simulink model "sampleModel1857_1_sub_sub"  (R2023a)
settings: Solver=VariableStepAuto  StartTime=0.0  StopTime=10.0  RelTol=1e-3
libraries: hdlsllib x4, simulink x2
settings Model: Creator=user1  LastModifiedBy=user1

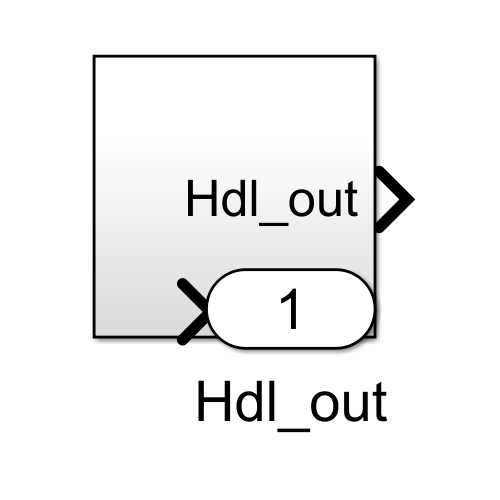
[thumbnail: Simulink's stored preview of the top-level diagram]
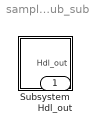
== system sampleModel1857_1_sub_sub ==
  Subsystem : Subsystem
  Hdl_out : Outport  OutDataTypeStr=uint8

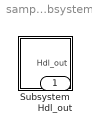
== system sampleModel1857_1_sub_sub/Subsystem ==
  Subsystem : Subsystem
  Hdl_out : Outport  OutDataTypeStr=uint8

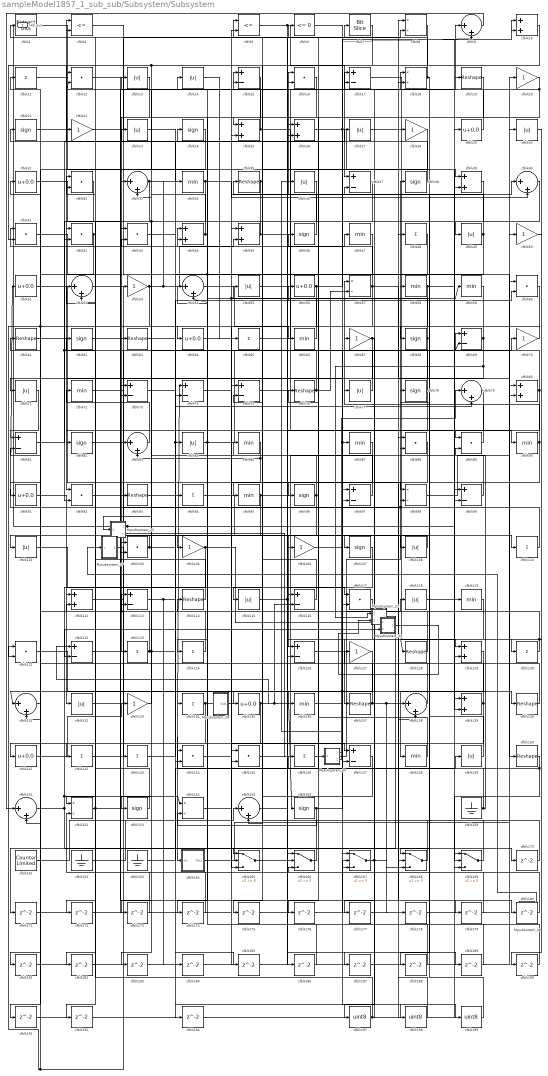
== system sampleModel1857_1_sub_sub/Subsystem/Subsystem ==
  Mysubsystem_10 : Subsystem  TreatAsAtomicUnit=on  RTWFcnName=Mysubsystem_10
      settings: RTWFcnNameOpts=User specified  RTWFileNameOpts=Use function name
  Mysubsystem_22 : Subsystem  TreatAsAtomicUnit=on  RTWFcnName=Mysubsystem_22
      settings: RTWFcnNameOpts=User specified  RTWFileNameOpts=Use function name
  Mysubsystem_23 : Subsystem  TreatAsAtomicUnit=on  RTWFcnName=Mysubsystem_23
      settings: RTWFcnNameOpts=User specified  RTWFileNameOpts=Use function name
  Mysubsystem_31 : Subsystem  TreatAsAtomicUnit=on  RTWFcnName=Mysubsystem_31
      settings: RTWFcnNameOpts=User specified  RTWFileNameOpts=Use function name
  Mysubsystem_37 : Subsystem  TreatAsAtomicUnit=on  RTWFcnName=Mysubsystem_37
      settings: RTWFcnNameOpts=User specified  RTWFileNameOpts=Use function name
  Mysubsystem_39 : Subsystem  TreatAsAtomicUnit=on  RTWFcnName=Mysubsystem_39
      settings: RTWFcnNameOpts=User specified  RTWFileNameOpts=Use function name
  Mysubsystem_40 : Subsystem  TreatAsAtomicUnit=on  RTWFcnName=Mysubsystem_40
      settings: RTWFcnNameOpts=User specified  RTWFileNameOpts=Use function name
  cfblk1 : simulink/Logic and Bit Operations/Extract Bits  bitsToExtract=Upper half  numBits=8  bitIdxRange=[0 7]  outScalingMode=Preserve fixed-point scaling
      settings: LibrarySourceBlock=|
      | hdlsllib/Logic and Bit
      | Operations/Extract Bits
  cfblk{10,25..26,39,44..45,80,112,129,139} (10 alike) : Sum  OutDataTypeStr=uint8
  cfblk{13..14,23,27,30,36,49,55,71,77,84,101,108,115,118,132,149} (17 alike) : Abs  OutDataTypeStr=uint8  SaturateOnIntegerOverflow=off
  cfblk{12,16,32,41..43,60,88..89,92,103,117,121,144..145} (15 alike) : DotProduct  OutDataTypeStr=uint8
  cfblk{20,22,28,50,53,67,70,104,106,127,133} (11 alike) : Gain  OutDataTypeStr=uint8
  cfblk{21,24,38,46,62,68,78,82,96,107,153,156} (12 alike) : Signum
  cfblk{11,48,65,94,110,123..124,130,134,142..143,146} (12 alike) : Sum  Inputs=+  OutDataTypeStr=uint8
  cfblk{15,17,37,69,73..75,81,97,99,113,116,122,126,147} (15 alike) : Sum  Inputs=+-  OutDataTypeStr=uint8
  cfblk{19,35,61,63,76,93,114,128,137,140,150} (11 alike) : Reshape
  cfblk{34,47,58..59,66,72,85,87,90,95,119,136,148} (13 alike) : MinMax  OutDataTypeStr=uint8
  cfblk{9,33,40,52,54,79,83,131,138,151,155} (11 alike) : Sum  Inputs=|++  OutDataTypeStr=uint8
  cfblk{29,31,51,56,64,91,135,141} (8 alike) : Bias  Bias=0.0  SaturateOnIntegerOverflow=off
  cfblk{8,18,57,98,152,154} (6 alike) : Product  Inputs=*/  OutDataTypeStr=uint8  RndMeth=Zero  SaturateOnIntegerOverflow=on
  cfblk159 : Ground
  cfblk161 : hdlsllib/Sources/Counter Limited  uplimit=7  tsamp=-1
  cfblk162 : Ground
  cfblk163 : Ground
  cfblk164 : Subsystem
      settings: LibrarySourceBlock=|
      | hdlsllib/Ports &
      | Subsystems/Subsystem
  cfblk{165..169} (5 alike) : Switch  OutDataTypeStr=uint8  SaturateOnIntegerOverflow=off  InputSameDT=off
  cfblk{170..192,194} (24 alike) : Delay  SampleTime=1
  cfblk197 : DataTypeConversion  OutDataTypeStr=uint8  SaturateOnIntegerOverflow=off  RndMeth=Floor
  cfblk198 : DataTypeConversion  OutDataTypeStr=uint8  SaturateOnIntegerOverflow=off  RndMeth=Floor
  cfblk199 : DataTypeConversion  OutDataTypeStr=uint8  SaturateOnIntegerOverflow=off  RndMeth=Floor
  cfblk2 : RelationalOperator  Operator=<=  OutDataTypeStr=boolean  InputSameDT=off
  cfblk5 : RelationalOperator  Operator=<=  OutDataTypeStr=boolean  InputSameDT=off
  cfblk6 : hdlsllib/Logic and Bit Operations/Compare To Zero  relop=<=  OutDataTypeStr=uint8
  cfblk7 : hdlsllib/Logic and Bit Operations/Bit Slice  lidx=7  ridx=0
  Hdl_out : Outport  OutDataTypeStr=uint8
  wires:
  Mysubsystem_40/1(Out1) -> Mysubsystem_37/1(u)
  Mysubsystem_39/1(Out1) -> cfblk122/1
  Mysubsystem_37/1(Out1) -> cfblk121/1, cfblk11/1
  Mysubsystem_31/1(Out1) -> Mysubsystem_22/2(In2)
  Mysubsystem_23/2(y) -> Mysubsystem_10/1(In1)
  Mysubsystem_23/1(Out1) -> cfblk129/2, Hdl_out/1
  Mysubsystem_22/1(Out1) -> cfblk171/1
  Mysubsystem_10/2(Out2) -> cfblk79/1
  Mysubsystem_10/1(Out1) -> cfblk36/1
  cfblk199/1 -> cfblk88/2
  cfblk198/1 -> cfblk88/1
  cfblk23/1 -> cfblk198/1
  cfblk197/1 -> cfblk22/1, cfblk127/1
  cfblk194/1 -> cfblk28/1
  cfblk63/1 -> cfblk194/1
  cfblk192/1 -> cfblk169/1
  cfblk191/1 -> cfblk138/2
  cfblk190/1 -> cfblk99/1
  cfblk50/1 -> cfblk190/1
  cfblk189/1 -> cfblk54/1
  cfblk106/1 -> cfblk189/1
  cfblk188/1 -> cfblk75/1
  cfblk187/1 -> cfblk18/2
  cfblk186/1 -> cfblk166/1
  cfblk165/1 -> cfblk186/1
  cfblk185/1 -> cfblk26/2
  cfblk184/1 -> cfblk25/2
  cfblk183/1 -> cfblk169/3
  cfblk182/1 -> cfblk45/1
  cfblk79/1 -> cfblk182/1
  cfblk181/1 -> cfblk60/1
  cfblk180/1 -> cfblk152/2
  cfblk179/1 -> cfblk166/3
  cfblk12/1 -> cfblk179/1
  cfblk178/1 -> cfblk39/2
  cfblk177/1 -> cfblk17/2
  cfblk176/1 -> cfblk167/2
  cfblk175/1 -> cfblk80/1
  cfblk147/1 -> cfblk175/1
  cfblk174/1 -> cfblk2/2
  cfblk173/1 -> cfblk52/1
  cfblk172/1 -> cfblk73/2
  cfblk171/1 -> cfblk145/1
  cfblk170/1 -> cfblk1/1
  cfblk74/1 -> cfblk170/1
  cfblk7/1 -> cfblk155/2
  cfblk116/1 -> cfblk15/1
  cfblk93/1 -> cfblk98/1
  cfblk85/1 -> cfblk145/2, cfblk83/2
  cfblk99/1 -> cfblk78/1
  cfblk161/1 -> cfblk5/2
  cfblk167/1 -> cfblk67/1, cfblk178/1
  cfblk76/1 -> cfblk55/1, cfblk57/2
  cfblk69/1 -> Mysubsystem_22/1(In1), cfblk191/1, cfblk68/1
  cfblk34/1 -> cfblk74/2, cfblk40/2
  cfblk67/1 -> cfblk176/1, cfblk177/1
  cfblk56/1 -> cfblk10/2, cfblk165/2
  cfblk18/1 -> cfblk5/1, cfblk168/1
  cfblk30/1 -> cfblk130/1
  cfblk124/1 -> cfblk31/1, cfblk113/1
  cfblk10/1 -> cfblk33/1, cfblk41/2
  cfblk80/1 -> cfblk13/1, cfblk172/1
  cfblk101/1 -> cfblk117/1
  cfblk81/1 -> cfblk27/1, cfblk69/2
  cfblk83/1 -> cfblk62/1
  cfblk132/1 -> cfblk83/1
  cfblk39/1 -> cfblk49/1
  cfblk87/1 -> cfblk165/1
  cfblk113/1 -> cfblk184/1, cfblk185/1
  cfblk152/1 -> cfblk73/1, cfblk192/1
  cfblk60/1 -> cfblk104/1
  cfblk48/1 -> cfblk144/2, cfblk174/1
  cfblk140/1 -> cfblk61/1
  cfblk151/1 -> Mysubsystem_31/2(In2), cfblk154/1, cfblk165/3
  cfblk19/1 -> cfblk103/2
  cfblk1/1 -> cfblk39/1
  cfblk54/1 -> cfblk106/1
  cfblk164/1(Out1) -> cfblk50/1
  cfblk37/1 -> cfblk42/2
  cfblk77/1 -> cfblk46/1
  cfblk38/1 -> cfblk2/1
  cfblk73/1 -> cfblk60/2
  cfblk131/1 -> cfblk81/2
  cfblk115/1 -> cfblk7/1, cfblk168/2
  cfblk61/1 -> cfblk167/1
  cfblk127/1 -> cfblk131/1, cfblk147/2
  cfblk58/1 -> cfblk10/1, cfblk71/1
  cfblk28/1 -> cfblk135/1
  cfblk46/1 -> cfblk35/1
  cfblk108/1 -> cfblk103/1
  cfblk154/1 -> cfblk59/1, cfblk40/1
  cfblk144/1 -> cfblk147/1
  cfblk78/1 -> cfblk153/1, cfblk24/1
  cfblk122/1 -> cfblk17/1
  cfblk138/1 -> cfblk6/1
  cfblk15/1 -> cfblk64/1
  cfblk133/1 -> cfblk23/1
  cfblk32/1 -> cfblk92/2
  cfblk68/1 -> cfblk21/1, cfblk167/3
  cfblk71/1 -> cfblk81/1
  cfblk29/1 -> cfblk19/1
  cfblk47/1 -> cfblk116/1
  cfblk36/1 -> Mysubsystem_23/1(In1), cfblk113/2
  cfblk42/1 -> cfblk112/1, cfblk181/1
  cfblk141/1 -> cfblk133/1
  cfblk112/1 -> cfblk48/1
  cfblk72/1 -> cfblk30/1
  cfblk92/1 -> cfblk136/1
  cfblk166/1 -> cfblk41/1
  cfblk25/1 -> cfblk150/1, cfblk15/2
  cfblk136/1 -> cfblk140/1
  cfblk123/1 -> cfblk79/2, cfblk183/1, cfblk32/2
  cfblk2/1 -> cfblk99/2
  cfblk168/1 -> cfblk44/2
  cfblk143/1 -> cfblk56/1
  cfblk53/1 -> cfblk121/2, cfblk91/1, cfblk45/2, cfblk34/1
  cfblk118/1 -> cfblk139/1
  cfblk16/1 -> cfblk25/1
  cfblk41/1 -> cfblk53/1
  cfblk163/1 -> cfblk146/1
  cfblk35/1 -> cfblk115/1, cfblk134/1
  cfblk20/1 -> cfblk96/1, cfblk12/2
  cfblk82/1 -> cfblk97/2
  cfblk103/1 -> cfblk101/1, cfblk117/2
  cfblk59/1 -> cfblk124/1
  cfblk153/1 -> cfblk72/1
  cfblk88/1 -> cfblk197/1
  cfblk64/1 -> cfblk108/1
  cfblk156/1 -> cfblk70/1, cfblk154/2
  cfblk6/1 -> cfblk87/1, cfblk199/1
  cfblk149/1 -> cfblk37/2
  cfblk11/1 -> cfblk143/1
  cfblk65/1 -> cfblk9/1
  cfblk44/1 -> cfblk144/1, cfblk12/1
  cfblk70/1 -> cfblk63/1
  cfblk62/1 -> cfblk138/1
  cfblk22/1 -> cfblk8/2
  cfblk130/1 -> cfblk52/2, cfblk128/1
  cfblk121/1 -> cfblk164/1(In1)
  cfblk13/1 -> cfblk93/1
  cfblk45/1 -> cfblk97/1, cfblk43/1
  cfblk31/1 -> cfblk123/1
  cfblk119/1 -> cfblk166/2
  cfblk137/1 -> cfblk168/3, cfblk180/1, cfblk75/2
  cfblk169/1 -> cfblk85/1
  cfblk162/1 -> cfblk155/1
  cfblk97/1 -> cfblk44/1
  cfblk155/1 -> cfblk149/1
  cfblk57/1 -> cfblk80/2, cfblk43/2, cfblk131/2
  cfblk40/1 -> cfblk82/1
  cfblk75/1 -> cfblk90/1
  cfblk129/1 -> cfblk148/1
  cfblk21/1 -> cfblk94/1
  cfblk98/1 -> cfblk20/1
  cfblk26/1 -> cfblk119/1, cfblk9/2
  cfblk134/1 -> cfblk151/2, cfblk18/1
  cfblk9/1 -> cfblk151/1
  cfblk84/1 -> cfblk29/1, cfblk54/2
  cfblk90/1 -> cfblk77/1, cfblk188/1
  cfblk139/1 -> cfblk112/2, cfblk173/1
  cfblk107/1 -> cfblk126/2
  cfblk117/1 -> cfblk137/1
  cfblk51/1 -> cfblk95/1
  cfblk95/1 -> cfblk152/1, cfblk47/1
  cfblk91/1 -> cfblk132/1
  cfblk27/1 -> cfblk8/1
  cfblk96/1 -> cfblk126/1, cfblk33/2
  cfblk89/1 -> cfblk57/1
  cfblk146/1 -> cfblk58/1
  cfblk94/1 -> cfblk107/1
  cfblk114/1 -> cfblk32/1
  cfblk43/1 -> cfblk84/1, cfblk139/2
  cfblk24/1 -> cfblk141/1
  cfblk5/1 -> cfblk37/1, cfblk187/1
  cfblk104/1 -> Mysubsystem_31/1(In1), cfblk122/2
  cfblk135/1 -> cfblk156/1, cfblk116/2, cfblk142/1
  cfblk66/1 -> cfblk14/1
  cfblk52/1 -> cfblk110/1
  cfblk110/1 -> cfblk51/1, cfblk98/2
  cfblk49/1 -> cfblk16/2, cfblk66/1
  cfblk148/1 -> cfblk76/1
  cfblk142/1 -> cfblk69/1
  cfblk145/1 -> cfblk38/1
  cfblk128/1 -> cfblk114/1
  cfblk159/1 -> cfblk16/1, cfblk89/2
  cfblk55/1 -> cfblk89/1
  cfblk8/1 -> cfblk42/1
  cfblk126/1 -> cfblk118/1
  cfblk150/1 -> cfblk74/1, cfblk169/2
  cfblk33/1 -> cfblk92/1, cfblk26/1
  cfblk17/1 -> cfblk129/1
  cfblk14/1 -> cfblk65/1

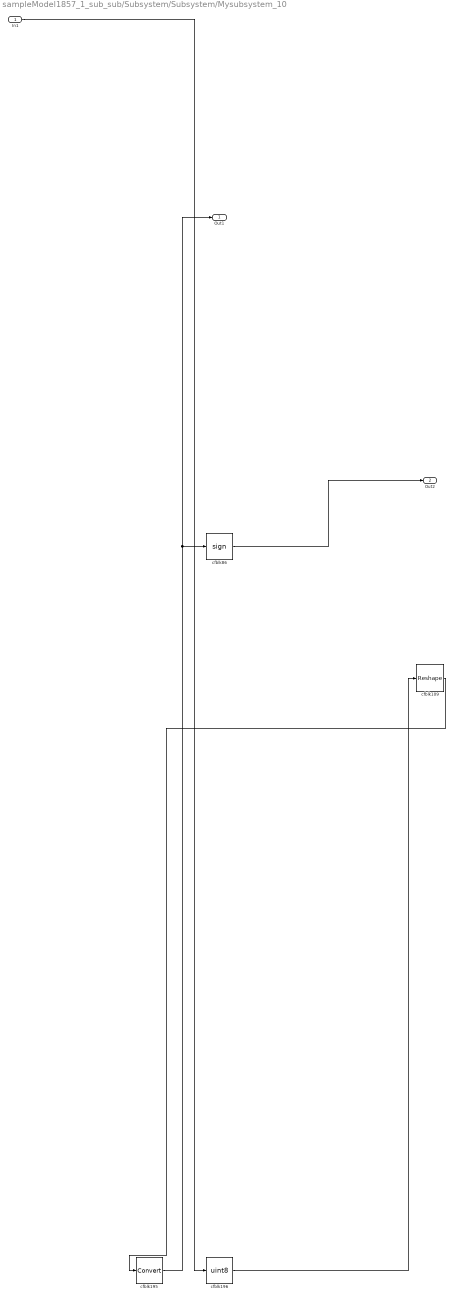
== system sampleModel1857_1_sub_sub/Subsystem/Subsystem/Mysubsystem_10 ==
  In1 : Inport
  cfblk109 : Reshape
  cfblk195 : DataTypeConversion  SaturateOnIntegerOverflow=off  RndMeth=Floor
  cfblk196 : DataTypeConversion  OutDataTypeStr=uint8  SaturateOnIntegerOverflow=off  RndMeth=Floor
  cfblk86 : Signum
  Out1 : Outport
  Out2 : Outport  Port=2
  wires:
  cfblk86/1 -> Out2/1
  cfblk109/1 -> cfblk195/1
  cfblk195/1 -> Out1/1, cfblk86/1
  cfblk196/1 -> cfblk109/1
  In1/1 -> cfblk196/1

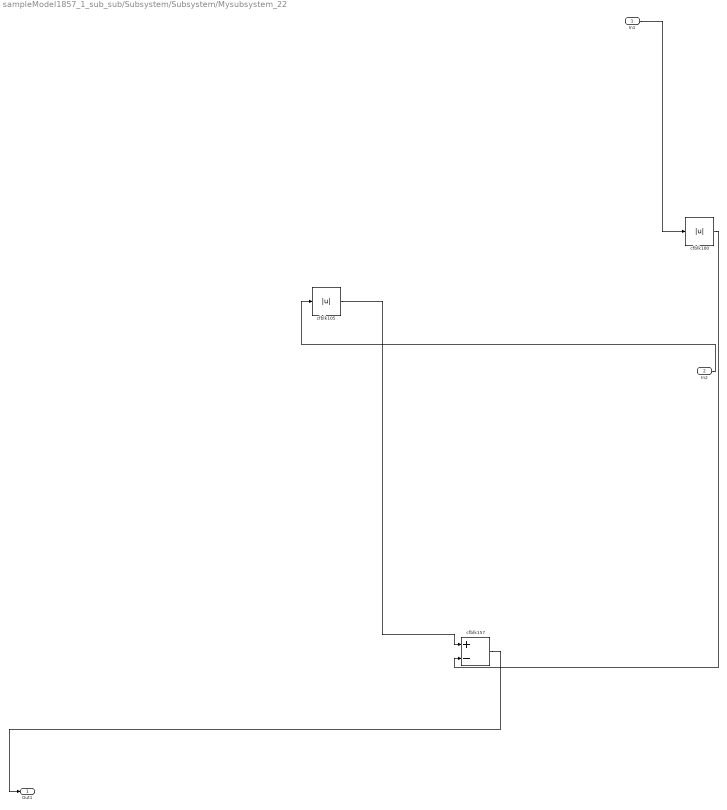
== system sampleModel1857_1_sub_sub/Subsystem/Subsystem/Mysubsystem_22 ==
  In1 : Inport
  In2 : Inport  Port=2
  cfblk100 : Abs  SaturateOnIntegerOverflow=off
  cfblk105 : Abs  SaturateOnIntegerOverflow=off
  cfblk157 : Sum  Inputs=+-
  Out1 : Outport
  wires:
  cfblk105/1 -> cfblk157/1
  In2/1 -> cfblk105/1
  cfblk100/1 -> cfblk157/2
  cfblk157/1 -> Out1/1
  In1/1 -> cfblk100/1

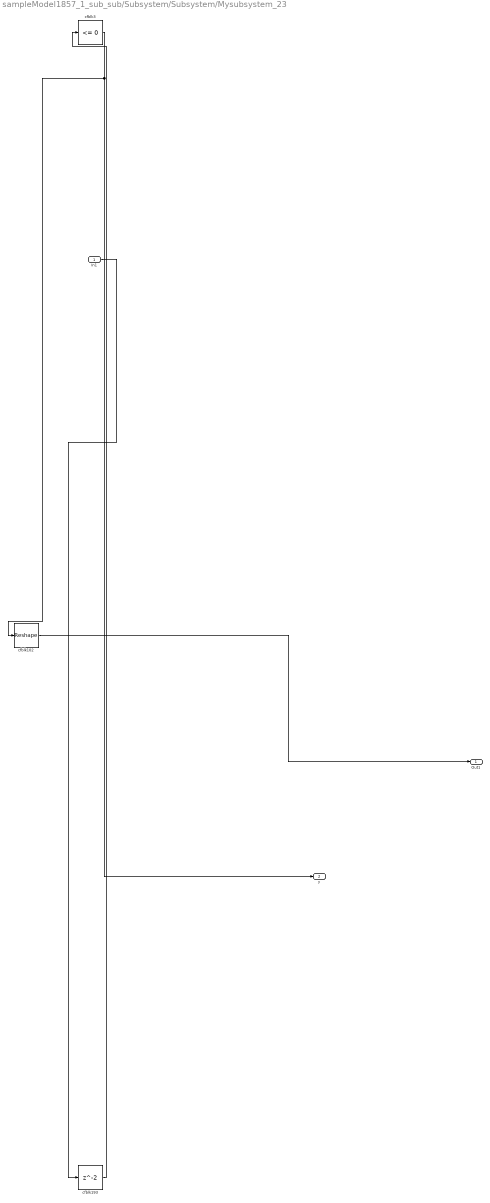
== system sampleModel1857_1_sub_sub/Subsystem/Subsystem/Mysubsystem_23 ==
  In1 : Inport
  cfblk102 : Reshape
  cfblk193 : Delay  SampleTime=1
  cfblk3 : hdlsllib/Logic and Bit Operations/Compare To Zero  relop=<=  OutDataTypeStr=boolean
  Out1 : Outport
  y : Outport  Port=2
  wires:
  cfblk193/1 -> cfblk3/1
  cfblk3/1 -> y/1, cfblk102/1
  cfblk102/1 -> Out1/1
  In1/1 -> cfblk193/1

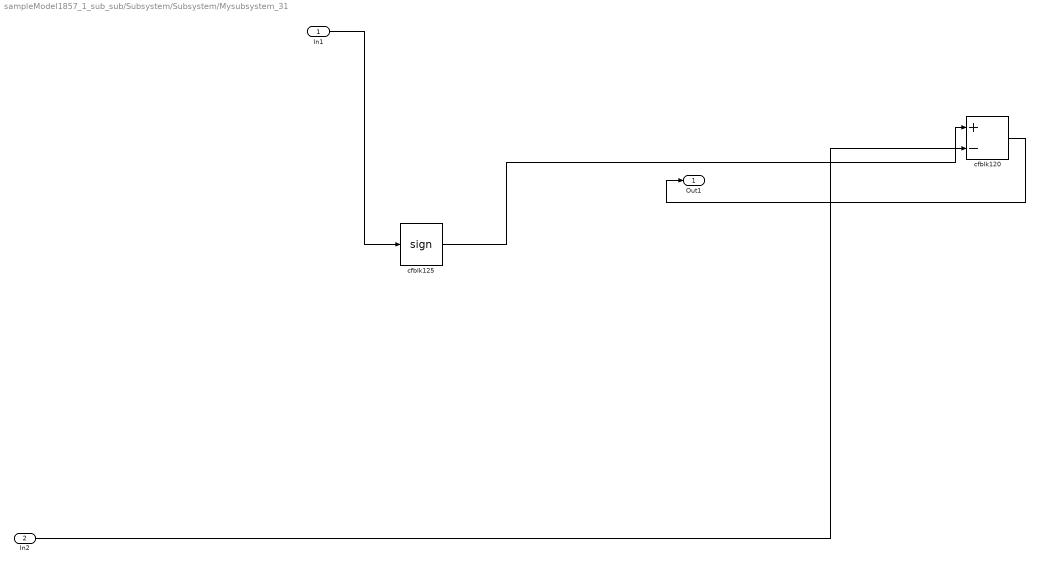
== system sampleModel1857_1_sub_sub/Subsystem/Subsystem/Mysubsystem_31 ==
  In1 : Inport
  In2 : Inport  Port=2
  cfblk120 : Sum  Inputs=+-
  cfblk125 : Signum
  Out1 : Outport
  wires:
  cfblk125/1 -> cfblk120/1
  In2/1 -> cfblk120/2
  In1/1 -> cfblk125/1
  cfblk120/1 -> Out1/1

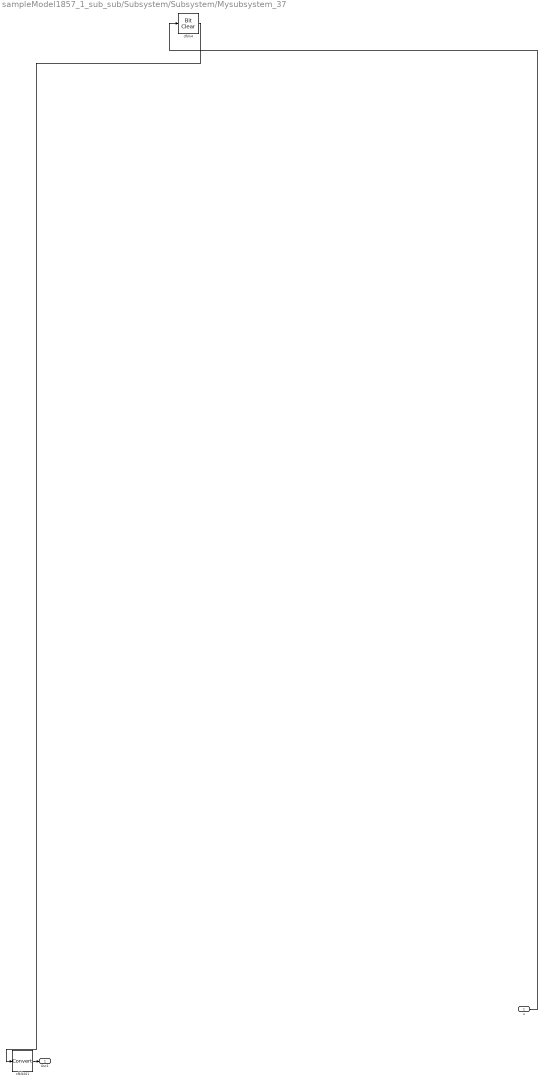
== system sampleModel1857_1_sub_sub/Subsystem/Subsystem/Mysubsystem_37 ==
  u : Inport
  cfblk201 : DataTypeConversion  SaturateOnIntegerOverflow=off  RndMeth=Floor
  cfblk4 : simulink/Logic and Bit Operations/Bit Clear  iBit=0
      settings: LibrarySourceBlock=|
      | hdlsllib/Logic and Bit
      | Operations/Bit Clear
  Out1 : Outport
  wires:
  cfblk201/1 -> Out1/1
  cfblk4/1 -> cfblk201/1
  u/1 -> cfblk4/1

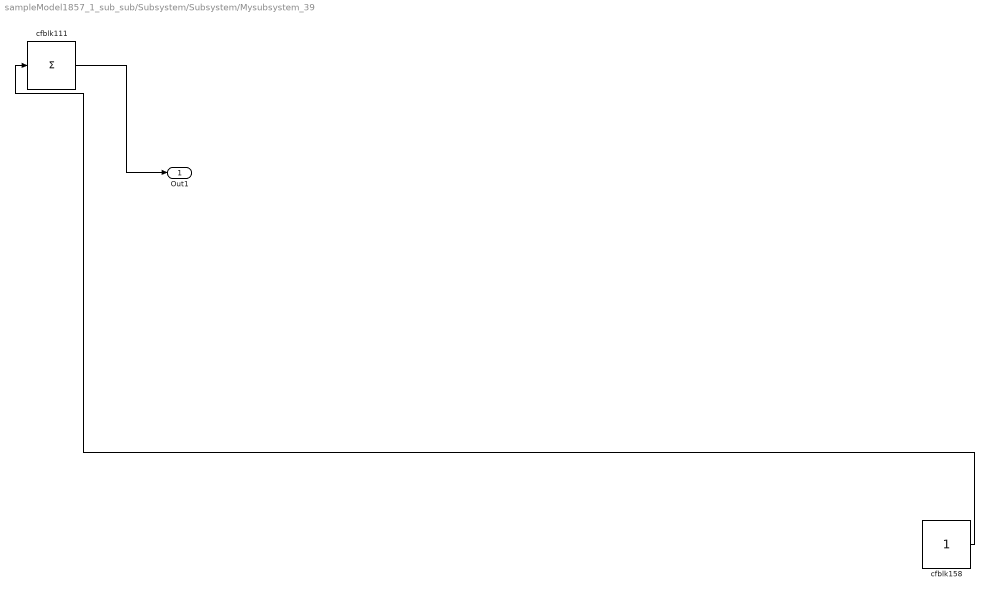
== system sampleModel1857_1_sub_sub/Subsystem/Subsystem/Mysubsystem_39 ==
  cfblk111 : Sum  Inputs=+
  cfblk158 : Constant  SampleTime=-1
  Out1 : Outport
  wires:
  cfblk111/1 -> Out1/1
  cfblk158/1 -> cfblk111/1

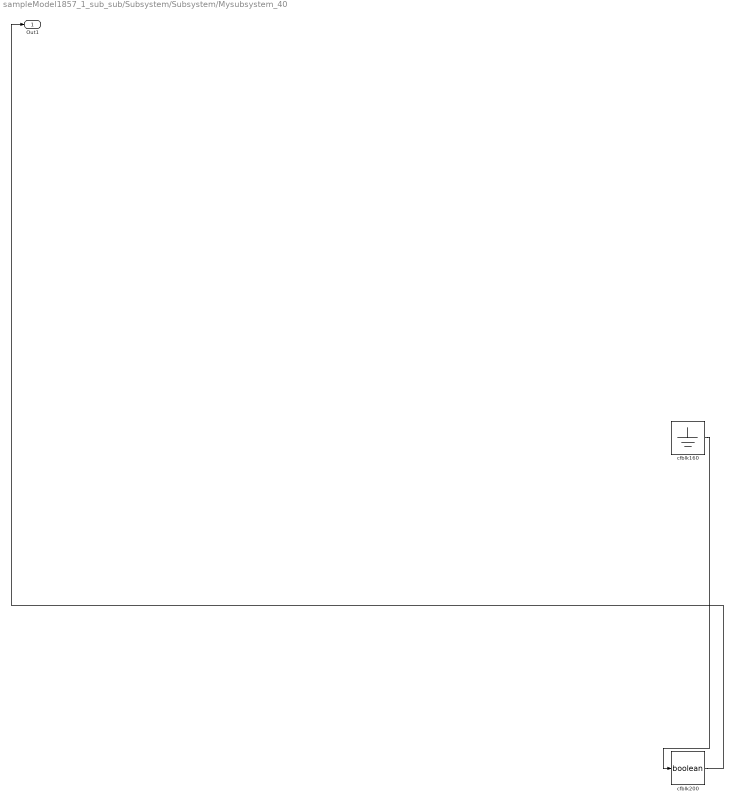
== system sampleModel1857_1_sub_sub/Subsystem/Subsystem/Mysubsystem_40 ==
  cfblk160 : Ground
  cfblk200 : DataTypeConversion  OutDataTypeStr=boolean  SaturateOnIntegerOverflow=off  RndMeth=Floor
  Out1 : Outport
  wires:
  cfblk160/1 -> cfblk200/1
  cfblk200/1 -> Out1/1

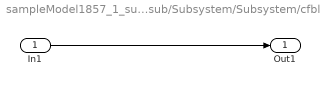
== system sampleModel1857_1_sub_sub/Subsystem/Subsystem/cfblk164 ==
  In1 : Inport
  Out1 : Outport
  wires:
  In1/1 -> Out1/1
